simulink model "InvDynOP"  (R2021a)
settings: Solver=FixedStepAuto  StartTime=0.0  StopTime=10.0  FixedStep=0.001  RelTol=1e-3
values from neighbouring files (symbols this model uses):
  kd = 2*z*w    [params.m]
  kp = w^2    [params.m]
settings Model: Creator=antoninoparisi  LastModifiedBy=antoninoparisi

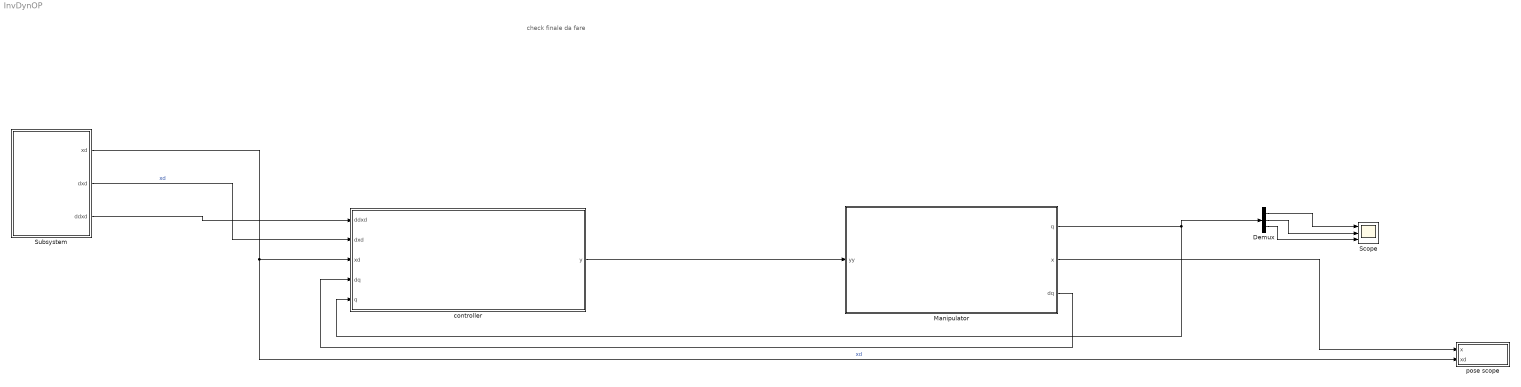
== system InvDynOP ==
  note: check finale da fare
  Demux : Demux  Outputs=3
  Manipulator : Subsystem
  Scope : Scope  NumInputPorts=3
  Subsystem : Subsystem
  controller : Subsystem
  pose scope : Subsystem
  wires:
  Manipulator/1(q) -> controller/5(q), Demux/1
  Manipulator/3(dq) -> controller/4(dq)
  Manipulator/2(x) -> pose scope/1(x)
  Subsystem/2(dxd) -> controller/2(dxd)  "xd"
  Subsystem/3(ddxd) -> controller/1(ddxd)
  Subsystem/1(xd) -> pose scope/2(xd), controller/3(xd)  "xd"
  controller/1(y) -> Manipulator/1(yy)
  Demux/1 -> Scope/1
  Demux/2 -> Scope/2
  Demux/3 -> Scope/3

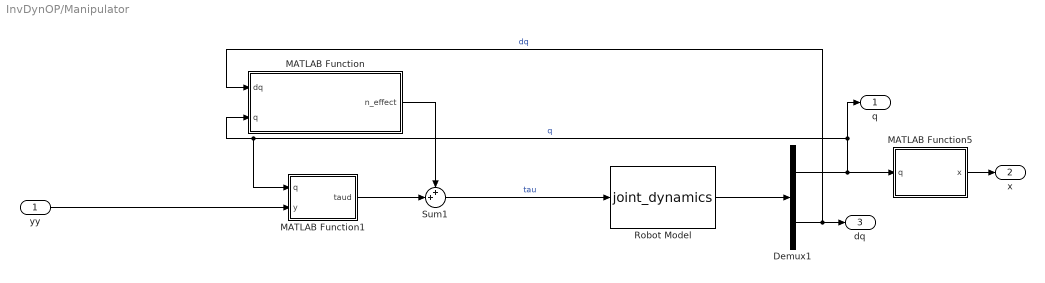
== system InvDynOP/Manipulator ==
  yy : Inport
  Demux1 : Demux  Outputs=[3, 3]
  MATLAB Function : MATLAB Function  TreatAsAtomicUnit=on
  MATLAB Function1 : MATLAB Function  TreatAsAtomicUnit=on
  MATLAB Function5 : MATLAB Function  TreatAsAtomicUnit=on
  Robot Model : S-Function  FunctionName=joint_dynamics  Parameters=robot  SFunctionDeploymentMode=off  EnableBusSupport=off
  Sum1 : Sum  Inputs=++|
  q : Outport
  x : Outport  Port=2
  dq : Outport  Port=3
  wires:
  Robot Model/1 -> Demux1/1
  Demux1/1 -> MATLAB Function5/1(q), q/1, MATLAB Function1/1(q), MATLAB Function/2(q)  "q"
  MATLAB Function5/1(x) -> x/1
  MATLAB Function1/1(taud) -> Sum1/2
  MATLAB Function/1(n_effect) -> Sum1/1
  Sum1/1 -> Robot Model/1  "tau"
  yy/1 -> MATLAB Function1/2(y)
  Demux1/2 -> MATLAB Function/1(dq), dq/1  "dq"

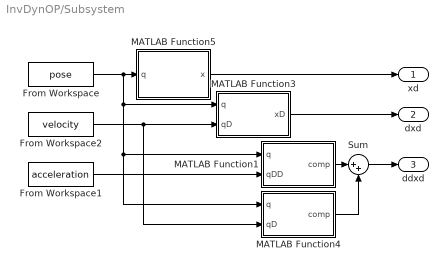
== system InvDynOP/Subsystem ==
  From Workspace : FromWorkspace  VariableName=pose
  From Workspace1 : FromWorkspace  VariableName=acceleration
  From Workspace2 : FromWorkspace  VariableName=velocity
  MATLAB Function1 : MATLAB Function  TreatAsAtomicUnit=on
  MATLAB Function3 : MATLAB Function  TreatAsAtomicUnit=on
  MATLAB Function4 : MATLAB Function  TreatAsAtomicUnit=on
  MATLAB Function5 : MATLAB Function  TreatAsAtomicUnit=on
  Sum : Sum  Inputs=|++
  xd : Outport
  dxd : Outport  Port=2
  ddxd : Outport  Port=3
  wires:
  From Workspace/1 -> MATLAB Function5/1(q), MATLAB Function3/1(q), MATLAB Function4/1(q), MATLAB Function1/1(q)
  Sum/1 -> ddxd/1
  From Workspace2/1 -> MATLAB Function4/2(qD), MATLAB Function3/2(qD)
  MATLAB Function4/1(comp) -> Sum/2
  From Workspace1/1 -> MATLAB Function1/2(qDD)
  MATLAB Function1/1(comp) -> Sum/1
  MATLAB Function3/1(xD) -> dxd/1
  MATLAB Function5/1(x) -> xd/1

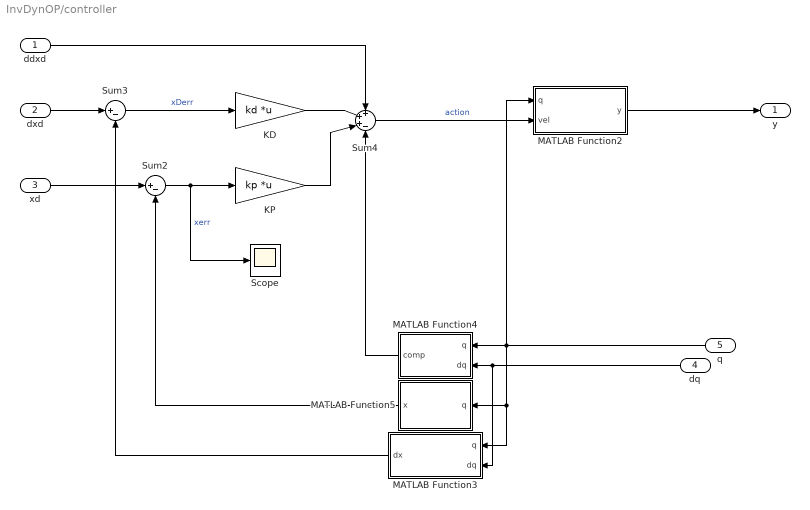
== system InvDynOP/controller ==
  ddxd : Inport
  dxd : Inport  Port=2
  xd : Inport  Port=3
  dq : Inport  Port=4
  q : Inport  Port=5
  KD : Gain  Gain=kd  Multiplication=Matrix(K*u) (u vector)
  KP : Gain  Gain=kp  Multiplication=Matrix(K*u) (u vector)
  MATLAB Function2 : MATLAB Function  TreatAsAtomicUnit=on
  MATLAB Function3 : MATLAB Function  TreatAsAtomicUnit=on
  MATLAB Function4 : MATLAB Function  TreatAsAtomicUnit=on
  MATLAB Function5 : MATLAB Function  TreatAsAtomicUnit=on
  Scope : Scope
  Sum2 : Sum  Inputs=|+-
  Sum3 : Sum  Inputs=|+-
  Sum4 : Sum  Inputs=+++-
  y : Outport
  wires:
  MATLAB Function2/1(y) -> y/1
  dxd/1 -> Sum3/1
  ddxd/1 -> Sum4/1
  xd/1 -> Sum2/1
  MATLAB Function3/1(dx) -> Sum3/2
  KP/1 -> Sum4/3
  Sum4/1 -> MATLAB Function2/2(vel)  "action"
  dq/1 -> MATLAB Function3/2(dq), MATLAB Function4/2(dq)
  q/1 -> MATLAB Function5/1(q), MATLAB Function3/1(q), MATLAB Function4/1(q), MATLAB Function2/1(q)
  Sum3/1 -> KD/1  "xDerr"
  MATLAB Function5/1(x) -> Sum2/2
  MATLAB Function4/1(comp) -> Sum4/4
  Sum2/1 -> KP/1, Scope/1  "xerr"
  KD/1 -> Sum4/2

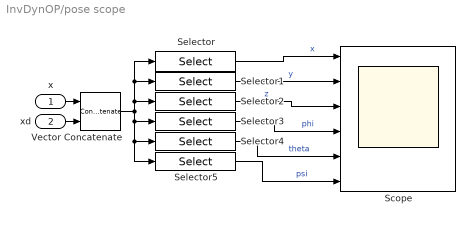
== system InvDynOP/pose scope ==
  x : Inport
  xd : Inport  Port=2
  Scope : Scope  NumInputPorts=6
  Selector : Selector  NumberOfDimensions=2  InputPortWidth=3  IndexOptions=Index vector (dialog),Select all  Indices=1,7  OutputSizes=6,6
  Selector1 : Selector  NumberOfDimensions=2  InputPortWidth=3  IndexOptions=Index vector (dialog),Select all  Indices=2,7  OutputSizes=6,6
  Selector2 : Selector  NumberOfDimensions=2  InputPortWidth=3  IndexOptions=Index vector (dialog),Select all  Indices=3,7  OutputSizes=6,6
  Selector3 : Selector  NumberOfDimensions=2  InputPortWidth=3  IndexOptions=Index vector (dialog),Select all  Indices=4,7  OutputSizes=6,6
  Selector4 : Selector  NumberOfDimensions=2  InputPortWidth=3  IndexOptions=Index vector (dialog),Select all  Indices=5,7  OutputSizes=6,6
  Selector5 : Selector  NumberOfDimensions=2  InputPortWidth=3  IndexOptions=Index vector (dialog),Select all  Indices=6,7  OutputSizes=6,6
  Vector Concatenate : Concatenate  Mode=Multidimensional array  ConcatenateDimension=2
  wires:
  x/1 -> Vector Concatenate/1
  xd/1 -> Vector Concatenate/2
  Selector1/1 -> Scope/2  "y"
  Selector5/1 -> Scope/6  "psi"
  Selector3/1 -> Scope/4  "phi"
  Selector/1 -> Scope/1  "x"
  Selector4/1 -> Scope/5  "theta"
  Vector Concatenate/1 -> Selector/1, Selector1/1, Selector2/1, Selector5/1, Selector4/1, Selector3/1
  Selector2/1 -> Scope/3  "z"

== matlab function InvDynOP/Subsystem/MATLAB Function3 ==
  data: q input; xD output; qD input
function xD = JA(q, qD)

xD = analyticalJacobian(q)*qD;

== matlab function InvDynOP/controller/MATLAB Function2 ==
  data: q input; y output; vel input
function y = JAinv(q, vel)

y = pinv(analyticalJacobian(q)) * vel;

== matlab function InvDynOP/controller/MATLAB Function3 ==
  data: q input; dx output; dq input
function dx = JA(q, dq)

dx = analyticalJacobian(q)*dq;

== matlab function InvDynOP/controller/MATLAB Function4 ==
  data: q input; comp output; dq input
function comp = JAD(q, dq)

t1 = q(1);
d1 = q(2);
t2 = q(3);

dt1 = dq(1);
dd1 = dq(2);
dt2 = dq(3);

a1 = 0.15;
a2 = 0.4;
a3 = 0.3;
a4 = 0.16;


J11 = a4*sin(t1)*sin(t2)*dt2 - a4*cos(t1)*cos(t2)*dt1 - a2*cos(t1)*dt1;
J13 = a4*sin(t1)*sin(t2)*dt1 - a4 * cos(t1)*cos(t2)*dt2;
J23 = -a4*sin(t2)*dt2;
J31 = -a2*sin(t1)*dt1 - a4*cos(t2)*sin(t1)*dt1 - a4 * cos(t1)*sin(t2)*dt2;
J33 = -a4 * cos(t1) * sin(t2) * dt1 - a4 * cos(t2)*sin(t1)*dt2;

JAD = zeros(6,3);

JAD(1,1) = J11;
JAD(1,3) = J13;
JAD(2,3) = J23;
JAD(3,1) = J31;
JAD(3,3) = J33;






comp = JAD*dq;

== matlab function InvDynOP/controller/MATLAB Function5 ==
  data: q input; x output
function x = K(q)

t1 = q(1);
d1 = q(2);
t2 = q(3);


a1 = 0.15;
a2 = 0.4;
a3 = 0.3;
a4 = 0.16;


% wrt frame 0
K = [[cos(t1)*cos(t2), -cos(t1)*sin(t2), -sin(t1),      a2*cos(t1) + a4*cos(t1)*cos(t2)]
    [        sin(t2),          cos(t2),        0,                 a4*sin(t2) - d1 - a3]
    [cos(t2)*sin(t1), -sin(t1)*sin(t2),  cos(t1), a1 + a2*sin(t1) + a4*cos(t2)*sin(t1)]
    [              0,                0,        0,                                    1]];

pos = K(1:3, 4);
ori = rotm2eul(K(1:3,1:3), 'ZYZ')';

x = [pos; ori];

== matlab function InvDynOP/Manipulator/MATLAB Function ==
  data: dq input; q input; n_effect output size=3
function n_effect = n(dq, q)

n_effect = C_Lagrangian(q, dq)*dq + G_Lagrangian(q);

== matlab function InvDynOP/Manipulator/MATLAB Function1 ==
  data: q input; taud output size=3; y input
function taud = B(q, y)

taud = B_Lagrangian(q)*y;

== matlab function InvDynOP/Subsystem/MATLAB Function4 ==
  data: q input; comp output; qD input
function comp = JAD(q, qD)

t1 = q(1);
d1 = q(2);
t2 = q(3);

Dt1 = qD(1);
Dt2 = qD(2);
Dd3 = qD(3);

a1 = 0.15;
a2 = 0.4;
a3 = 0.3;
a4 = 0.16;


JAD = [[- a4*cos(t1 + t2) - (pi*cos(t1))/100, 0,        -a4*cos(t1 + t2)]
[                                   0, 0,             -a4*sin(t2)]
[- a4*sin(t1 + t2) - (pi*sin(t1))/100, 0,        -a4*sin(t1 + t2)]
[                                   0, 0,                       0]
[                                   0, 0,                       0]
[                                   0, 0, -2^(1/2)*sin(t1 + pi/4)]];
comp = JAD*qD;

== matlab function InvDynOP/Subsystem/MATLAB Function5 ==
  data: q input; x output
function x = K(q)

t1 = q(1);
d1 = q(2);
t2 = q(3);


a1 = 0.15;
a2 = 0.4;
a3 = 0.3;
a4 = 0.16;


% wrt frame 0
K = [[cos(t1)*cos(t2), -cos(t1)*sin(t2), -sin(t1),      a2*cos(t1) + a4*cos(t1)*cos(t2)]
    [        sin(t2),          cos(t2),        0,                 a4*sin(t2) - d1 - a3]
    [cos(t2)*sin(t1), -sin(t1)*sin(t2),  cos(t1), a1 + a2*sin(t1) + a4*cos(t2)*sin(t1)]
    [              0,                0,        0,                                    1]];

pos = K(1:3, 4);
ori = rotm2eul(K(1:3,1:3), 'ZYZ')';

x = [pos; ori];

== matlab function InvDynOP/Subsystem/MATLAB Function1 ==
  data: q input; comp output; qDD input
function comp = JA(q, qDD)

comp = analyticalJacobian(q)*qDD;

== matlab function InvDynOP/Manipulator/MATLAB Function5 ==
  data: q input; x output
function x = K(q)

t1 = q(1);
d1 = q(2);
t2 = q(3);


a1 = 0.15;
a2 = 0.4;
a3 = 0.3;
a4 = 0.16;


% wrt frame 0
K = [[cos(t1)*cos(t2), -cos(t1)*sin(t2), -sin(t1),      a2*cos(t1) + a4*cos(t1)*cos(t2)]
    [        sin(t2),          cos(t2),        0,                 a4*sin(t2) - d1 - a3]
    [cos(t2)*sin(t1), -sin(t1)*sin(t2),  cos(t1), a1 + a2*sin(t1) + a4*cos(t2)*sin(t1)]
    [              0,                0,        0,                                    1]];

pos = K(1:3, 4);
ori = rotm2eul(K(1:3,1:3), 'ZYZ')';

x = [pos; ori];
